simulink model "System_1"  (R2020a)
settings: Solver=FixedStepAuto  StartTime=0.0  StopTime=10.0  FixedStep=1  RelTol=1e-3
settings Model: Creator=NIKITA  LastModifiedBy=NIKITA
settings DataIOCC: SaveOutput=off  SaveTime=off

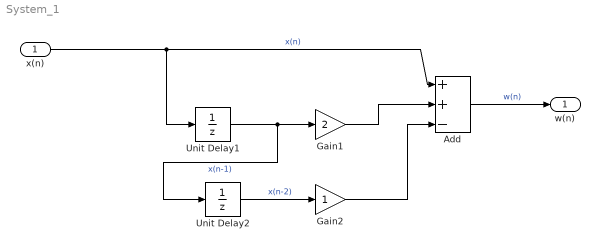
== system System_1 ==
  x(n) : Inport  OutDataTypeStr=double  PortDimensions=[1 1]  SampleTime=[1,0]
  Add : Sum  Inputs=++-
  Gain1 : Gain  Gain=2
  Gain2 : Gain
  Unit Delay1 : UnitDelay  SampleTime=-1  HasFrameUpgradeWarning=on
  Unit Delay2 : UnitDelay  SampleTime=-1  HasFrameUpgradeWarning=on
  w(n) : Outport  OutDataTypeStr=double  PortDimensions=[1 1]  SampleTime=[1,0]
  wires:
  Add/1 -> w(n)/1  "w(n)"
  Unit Delay1/1 -> Gain1/1, Unit Delay2/1  "x(n-1)"
  Gain1/1 -> Add/2
  x(n)/1 -> Unit Delay1/1, Add/1  "x(n)"
  Unit Delay2/1 -> Gain2/1  "x(n-2)"
  Gain2/1 -> Add/3
